simulink model "satsim"  (R2022b)
settings: Solver=VariableStepAuto  StartTime=0.0  StopTime=3600  RelTol=1e-3
InitFcn:
  | run data_initialize.m
StopFcn:
  | figure;
  | subplot(3,1,1);
  | plot(out.t,out.error_anles(:,1));
  | ylabel('yaw(deg)');
  | xlabel('simtime(s)');
  | 
  | subplot(3,1,2);
  | plot(out.t,out.error_anles(:,2));
  | ylabel('pitch(deg)');
  | xlabel('simtime(s)');
  | 
  | subplot(3,1,3);
  | plot(out.t,out.error_anles(:,3));
  | ylabel('roll(deg)');
  | xlabel('simtime(s)');
values from neighbouring files (symbols this model uses):
  Hb0 = IBd*Wb0    [data_initialize.m]
  IBd = [93,-0.07,0;-0.07,80,-0.03;0,-0.03,107]    [data_initialize.m]
  InvIBd = inv(IBd)    [data_initialize.m]
  miu = 398600.44e+9    (= 398600440000000)    [data_initialize.m]    (also in magnetic_Torque.m)
  Qb0 = [1;0;0;0]    [data_initialize.m]
  r0 = 1e+6*[-0.24322284327422;-3.79199144866264;6.32444994784559]    [data_initialize.m]
  T_orbit = 2*pi/Womag    [data_initialize.m]    (also in magnetic_Torque.m)
  v0 = 1e+3*[-1.64209188480826; 6.17220916529869; 3.63756062689151]    [data_initialize.m]
undefined symbols (not defined in the file or in its folder): magnetic_Torque
libraries: sharedutil x4, sharedtransform x2
settings Model: Creator=kuokc  LastModifiedBy=kuokc
settings DebuggingCC: UnderSpecifiedDimensionMsg=warning

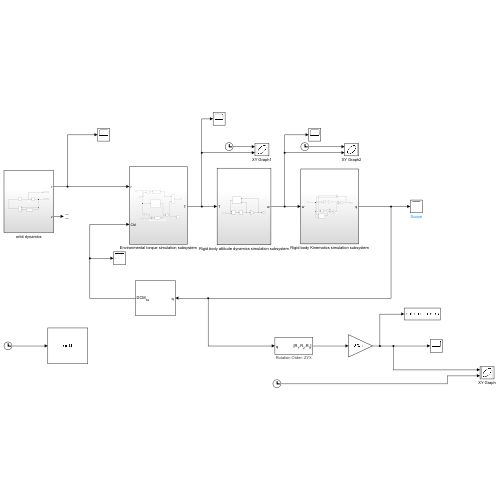
[thumbnail: Simulink's stored preview of the top-level diagram]
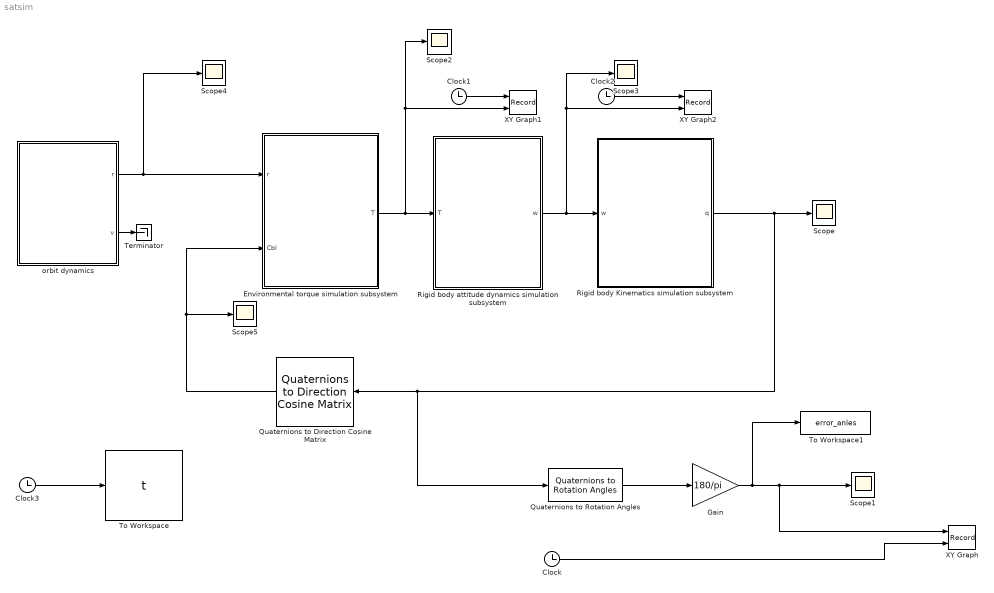
== system satsim ==
  Clock{,1..3} (4 alike) : Clock
  Environmental torque simulation subsystem : Subsystem
  Gain : Gain  Gain=180/pi
  Quaternions to Direction Cosine Matrix : sharedtransform/Quaternions to  Direction Cosine Matrix  aMode=aMode
      settings: LibrarySourceBlock=|
      | aerolibtransform2/Quaternions to
      | Direction Cosine Matrix
  Quaternions to Rotation Angles : sharedtransform/Quaternions to Rotation Angles  rotationOrder=ZYX  aMode=aMode
  Rigid body Kinematics simulation subsystem : Subsystem
  Rigid body attitude dynamics simulation subsystem : Subsystem
  Scope{,1..5} (6 alike) : Scope
  Terminator : Terminator
  To Workspace : ToWorkspace  VariableName=t  SampleTime=-1
  To Workspace1 : ToWorkspace  VariableName=error_anles  SampleTime=-1
  XY Graph : Record  FileSettingsInternal="{\"entries\":[{\"content\":{\"excelSettings\":{\"content\":{},\"type\":\"Streamout.ExcelSettings\"}},\"type\":\"Streamout.FileSettingStorage\",\"uuid\":\"d5935534-3018-4682-9264-9e126ec8adf6\"}],\"packageUris\":[\"http://schema.mathworks.com/mf0/streamout_blocks/R2020a\"],\"version\":\"1.0\"}"  Layout=[1 1]  SignalsInternal="{\"entries\":[{\"content\":{\"signals\":[{\"content\":{\"blockPath\":[\"satsim/XY Graph\"],\"channel\":[],\"dimensions\":[3],\"domain\":\"satsim/XY Graph\",\"hasChildren\":true,\"lineColor\":\"#fe330a\",\"plots\":[],\"port\":1,\"sid\":[\"\"],\"signalID\":166,\"signalName\":\"Gain\"},\"type\":\"RecordBlkView.Signal\",\"uuid\":\"ff8d8c7c-5dc9-4f5c-8804-467ea547fb30\"},{\"content\":{\"blockPath\":[\"satsim/XY Graph\"],\"channel\":[1],\"dimensions\":[3],\"domain\":\"satsim/XY Graph\",\"lineColor\":\"#ff6929\",\"parentID\":166,\"plots\":[1],\"port\":1,\"sid\":[\"\"],\"signalID\":167,\"signalName\":\"Gain\"},\"type\":\"RecordBlkView.Signal\",\"uuid\":\"aac24d3e-19aa-4daa-bfc7-aa7599c39485\"},{\"content\":{\"blockPath\":[\"satsim/XY Graph\"],\"channel\":[],\"dimensions\":[1],\"domain\":\"satsim/XY Graph\",\"lineColor\":\"#139fff\",\"plots\":[1],\"port\":2,\"sid\":[\"\"],\"signalID\":171,\"signalName\":\"Clock\"},\"type\":\"RecordBlkView.Signal\",\"uuid\":\"c5ea15f9-4ec4-4ccd-9c11-f3da415460d7\"},{\"content\":{\"blockPath\":[\"satsim/XY Graph\"],\"channel\":[2],\"dimensions\":[3],\"domain\":\"satsim/XY Graph\",\"lineColor\":\"#7e2f8e\",\"parentID\":166,\"plots\":[1],\"port\":1,\"sid\":[\"\"],\"signalID\":223,\"signalName\":\"Gain\"},\"type\":\"RecordBlkView.Signal\",\"uuid\":\"33786e91-945b-4266-af8d-a53b52915fa5\"},{\"content\":{\"blockPath\":[\"satsim/XY Graph\"],\"channel\":[3],\"dimensions\":[3],\"domain\":\"satsim/XY Graph\",\"lineColor\":\"#77ac30\",\"parentID\":166,\"plots\":[1],\"port\":1,\"sid\":[\"\"],\"signalID\":224,\"signalName\":\"Gain\"},\"type\":\"RecordBlkView.Signal\",\"uuid\":\"7c01fa1b-1002-497a-81b7-3edfb265aba0\"}]},\"type\":\"RecordBlkView.InputSignals\",\"uuid\":\"e2e14102-18f6-4548-bbad-20976a6fad0f\"}],\"packageUris\":[\"http://schema.mathworks.com/mf0/streamout_blocks/R2020a\"],\"version\":\"1.0\"}"  VisualizationBindings="{\"xyplotplugin\":{\"info\":[{\"series\":[{\"bindingParametersList\":[{\"parameter\":\"X-Axis\",\"signalID\":171,\"signalName\":\"Clock\"},{\"parameter\":\"Y-Axis\",\"signalID\":167,\"signalName\":\"Gain(1)\"}],\"seriesID\":65218},{\"bindingParametersList\":[{\"parameter\":\"X-Axis\",\"signalID\":171,\"signalName\":\"Clock\"},{\"parameter\":\"Y-Axis\",\"signalID\":223,\"signalName\":\"Gain(2)\"}],\"seriesID\":37351},{\"bindingParametersList\":[{\"parameter\":\"X-Axis\",\"signalID\":171,\"signalName\":\"Clock\"},{\"parameter\":\"Y-Axis\",\"signalID\":224,\"signalName\":\"Gain(3)\"}],\"seriesID\":18376}],\"subplotID\":1}]}}"  CompatibilityTag=XY
  XY Graph1 : Record  FileSettingsInternal="{\"entries\":[{\"content\":{\"excelSettings\":{\"content\":{},\"type\":\"Streamout.ExcelSettings\"}},\"type\":\"Streamout.FileSettingStorage\",\"uuid\":\"255aa934-7037-4e8a-b86c-47c5749866d0\"}],\"packageUris\":[\"http://schema.mathworks.com/mf0/streamout_blocks/R2020a\"],\"version\":\"1.0\"}"  Layout=[1 1]  SignalsInternal="{\"entries\":[{\"content\":{\"signals\":[{\"content\":{\"blockPath\":[\"satsim/XY Graph1\"],\"channel\":[],\"dimensions\":[1],\"domain\":\"satsim/XY Graph1\",\"lineColor\":\"#139fff\",\"plots\":[1],\"port\":1,\"sid\":[\"\"],\"signalID\":175,\"signalName\":\"Clock1\"},\"type\":\"RecordBlkView.Signal\",\"uuid\":\"f30088d5-5af3-48de-8442-de16e8626a94\"},{\"content\":{\"blockPath\":[\"satsim/XY Graph1\"],\"channel\":[],\"dimensions\":[3],\"domain\":\"satsim/XY Graph1\",\"hasChildren\":true,\"lineColor\":\"#edb120\",\"plots\":[],\"port\":2,\"sid\":[\"\"],\"signalID\":179,\"signalName\":\"Environmental torque simulation subsystem\"},\"type\":\"RecordBlkView.Signal\",\"uuid\":\"edce25b7-b2b4-4c0f-8394-da9e60d165bc\"},{\"content\":{\"blockPath\":[\"satsim/XY Graph1\"],\"channel\":[1],\"dimensions\":[3],\"domain\":\"satsim/XY Graph1\",\"lineColor\":\"#b746ff\",\"parentID\":179,\"plots\":[1],\"port\":2,\"sid\":[\"\"],\"signalID\":180,\"signalName\":\"Environmental torque simulation subsystem\"},\"type\":\"RecordBlkView.Signal\",\"uuid\":\"6268e222-72db-4a7c-9950-fb12145a70e4\"},{\"content\":{\"blockPath\":[\"satsim/XY Graph1\"],\"channel\":[2],\"dimensions\":[3],\"domain\":\"satsim/XY Graph1\",\"lineColor\":\"#4dbeee\",\"parentID\":179,\"plots\":[1],\"port\":2,\"sid\":[\"\"],\"signalID\":225,\"signalName\":\"Environmental torque simulation subsystem\"},\"type\":\"RecordBlkView.Signal\",\"uuid\":\"601717bb-ab46-42cc-a806-3aeeabde5761\"},{\"content\":{\"blockPath\":[\"satsim/XY Graph1\"],\"channel\":[3],\"dimensions\":[3],\"domain\":\"satsim/XY Graph1\",\"lineColor\":\"#a2142f\",\"parentID\":179,\"plots\":[1],\"port\":2,\"sid\":[\"\"],\"signalID\":226,\"signalName\":\"Environmental torque simulation subsystem\"},\"type\":\"RecordBlkView.Signal\",\"uuid\":\"82322a17-9809-4131-ba40-ba05a57ed190\"}]},\"type\":\"RecordBlkView.InputSignals\",\"uuid\":\"6b813904-0c0e-4fcd-a3f5-5389ecdd5549\"}],\"packageUris\":[\"http://schema.mathworks.com/mf0/streamout_blocks/R2020a\"],\"version\":\"1.0\"}"  VisualizationBindings="{\"xyplotplugin\":{\"info\":[{\"series\":[{\"bindingParametersList\":[{\"parameter\":\"X-Axis\",\"signalID\":175,\"signalName\":\"Clock1\"},{\"parameter\":\"Y-Axis\",\"signalID\":225,\"signalName\":\"Environmental torque simulation subsystem(2)\"}],\"seriesID\":232},{\"bindingParametersList\":[{\"parameter\":\"X-Axis\",\"signalID\":175,\"signalName\":\"Clock1\"},{\"parameter\":\"Y-Axis\",\"signalID\":180,\"signalName\":\"Environmental torque simulation subsystem(1)\"}],\"seriesID\":54442},{\"bindingParametersList\":[{\"parameter\":\"X-Axis\",\"signalID\":175,\"signalName\":\"Clock1\"},{\"parameter\":\"Y-Axis\",\"signalID\":226,\"signalName\":\"Environmental torque simulation subsystem(3)\"}],\"seriesID\":10841}],\"subplotID\":1}]}}"  CompatibilityTag=XY
  XY Graph2 : Record  FileSettingsInternal="{\"entries\":[{\"content\":{\"excelSettings\":{\"content\":{},\"type\":\"Streamout.ExcelSettings\"}},\"type\":\"Streamout.FileSettingStorage\",\"uuid\":\"a904b502-5531-4921-b81d-345613b13fcd\"}],\"packageUris\":[\"http://schema.mathworks.com/mf0/streamout_blocks/R2020a\"],\"version\":\"1.0\"}"  Layout=[1 1]  SignalsInternal="{\"entries\":[{\"content\":{\"signals\":[{\"content\":{\"blockPath\":[\"satsim/XY Graph2\"],\"channel\":[],\"dimensions\":[1],\"domain\":\"satsim/XY Graph2\",\"lineColor\":\"#139fff\",\"plots\":[1],\"port\":1,\"sid\":[\"\"],\"signalID\":184,\"signalName\":\"Clock2\"},\"type\":\"RecordBlkView.Signal\",\"uuid\":\"078e9baf-7ef4-4016-bcd0-3751340707a6\"},{\"content\":{\"blockPath\":[\"satsim/XY Graph2\"],\"channel\":[],\"dimensions\":[3],\"domain\":\"satsim/XY Graph2\",\"hasChildren\":true,\"lineColor\":\"#4dbeee\",\"plots\":[],\"port\":2,\"sid\":[\"\"],\"signalID\":188,\"signalName\":\"Rigid body attitude dynamics simulation subsystem\"},\"type\":\"RecordBlkView.Signal\",\"uuid\":\"c9ad4af1-ab2d-4e04-a6fb-069e0a9b0214\"},{\"content\":{\"blockPath\":[\"satsim/XY Graph2\"],\"channel\":[1],\"dimensions\":[3],\"domain\":\"satsim/XY Graph2\",\"lineColor\":\"#b746ff\",\"parentID\":188,\"plots\":[1],\"port\":2,\"sid\":[\"\"],\"signalID\":189,\"signalName\":\"Rigid body attitude dynamics simulation subsystem\"},\"type\":\"RecordBlkView.Signal\",\"uuid\":\"ffc096b0-7673-4870-9807-8de7d9d5d4a3\"},{\"content\":{\"blockPath\":[\"satsim/XY Graph2\"],\"channel\":[2],\"dimensions\":[3],\"domain\":\"satsim/XY Graph2\",\"lineColor\":\"#4dbeee\",\"parentID\":188,\"plots\":[1],\"port\":2,\"sid\":[\"\"],\"signalID\":227,\"signalName\":\"Rigid body attitude dynamics simulation subsystem\"},\"type\":\"RecordBlkView.Signal\",\"uuid\":\"53275a63-6ee4-490c-ab35-1f561b321303\"},{\"content\":{\"blockPath\":[\"satsim/XY Graph2\"],\"channel\":[3],\"dimensions\":[3],\"domain\":\"satsim/XY Graph2\",\"lineColor\":\"#a2142f\",\"parentID\":188,\"plots\":[1],\"port\":2,\"sid\":[\"\"],\"signalID\":228,\"signalName\":\"Rigid body attitude dynamics simulation subsystem\"},\"type\":\"RecordBlkView.Signal\",\"uuid\":\"53a253ef-b50a-41c3-8cb9-5fbddfddb443\"}]},\"type\":\"RecordBlkView.InputSignals\",\"uuid\":\"eac32adb-4985-4d46-95b6-7ca8e99f0a7e\"}],\"packageUris\":[\"http://schema.mathworks.com/mf0/streamout_blocks/R2020a\"],\"version\":\"1.0\"}"  VisualizationBindings="{\"xyplotplugin\":{\"info\":[{\"series\":[{\"bindingParametersList\":[{\"parameter\":\"X-Axis\",\"signalID\":184,\"signalName\":\"Clock2\"},{\"parameter\":\"Y-Axis\",\"signalID\":228,\"signalName\":\"Rigid body attitude dynamics simulation subsystem(3)\"}],\"seriesID\":16914},{\"bindingParametersList\":[{\"parameter\":\"X-Axis\",\"signalID\":184,\"signalName\":\"Clock2\"},{\"parameter\":\"Y-Axis\",\"signalID\":227,\"signalName\":\"Rigid body attitude dynamics simulation subsystem(2)\"}],\"seriesID\":8746},{\"bindingParametersList\":[{\"parameter\":\"X-Axis\",\"signalID\":184,\"signalName\":\"Clock2\"},{\"parameter\":\"Y-Axis\",\"signalID\":189,\"signalName\":\"Rigid body attitude dynamics simulation subsystem(1)\"}],\"seriesID\":5743}],\"subplotID\":1}]}}"  CompatibilityTag=XY
  orbit dynamics : Subsystem
  wires:
  Rigid body attitude dynamics simulation subsystem/1(w) -> XY Graph2/2, Scope3/1, Rigid body Kinematics simulation subsystem/1(w)
  Environmental torque simulation subsystem/1(T) -> XY Graph1/2, Scope2/1, Rigid body attitude dynamics simulation subsystem/1(T)
  orbit dynamics/2(v) -> Terminator/1
  Quaternions to Direction Cosine Matrix/1 -> Scope5/1, Environmental torque simulation subsystem/2(CbI)
  Rigid body Kinematics simulation subsystem/1(q) -> Quaternions to Rotation Angles/1, Quaternions to Direction Cosine Matrix/1, Scope/1
  Quaternions to Rotation Angles/1 -> Gain/1
  Gain/1 -> To Workspace1/1, XY Graph/1, Scope1/1
  Clock/1 -> XY Graph/2
  Clock1/1 -> XY Graph1/1
  Clock2/1 -> XY Graph2/1
  Clock3/1 -> To Workspace/1
  orbit dynamics/1(r) -> Scope4/1, Environmental torque simulation subsystem/1(r)

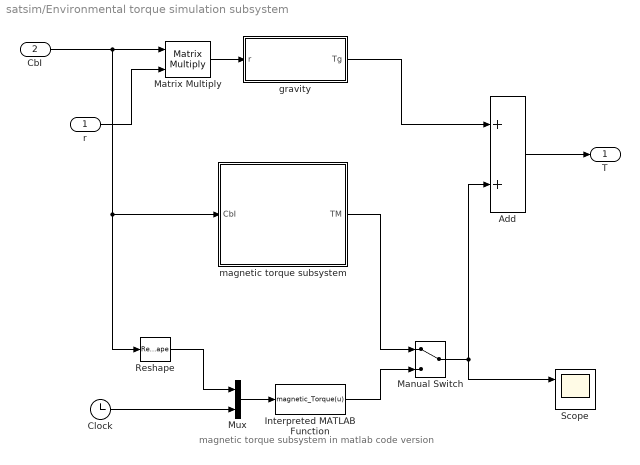
== system satsim/Environmental torque simulation subsystem ==
  note: magnetic torque subsystem in matlab code version
  r : Inport  PortDimensions=3
  CbI : Inport  Port=2
  " gravity" : Subsystem
  Add : Sum
  Clock : Clock
  Interpreted MATLAB Function : MATLABFcn  MATLABFcn=magnetic_Torque(u)  OutputDimensions=3
  Manual Switch : ManualSwitch
  Matrix Multiply : Product  Multiplication=Matrix(*)
  Mux : Mux  Inputs=2
  Reshape : Reshape
  Scope : Scope  NumInputPorts=2
  magnetic torque subsystem : Subsystem
  T : Outport
  wires:
  r/1 -> Matrix Multiply/2
  Matrix Multiply/1 -> " gravity"/1(r)
  " gravity"/1(Tg) -> Add/1
  Add/1 -> T/1
  CbI/1 -> Matrix Multiply/1, magnetic torque subsystem/1(CbI), Reshape/1
  Clock/1 -> Mux/2
  Reshape/1 -> Mux/1
  Mux/1 -> Interpreted MATLAB Function/1
  Interpreted MATLAB Function/1 -> Manual Switch/2
  Manual Switch/1 -> Add/2, Scope/1
  magnetic torque subsystem/1(TM) -> Manual Switch/1

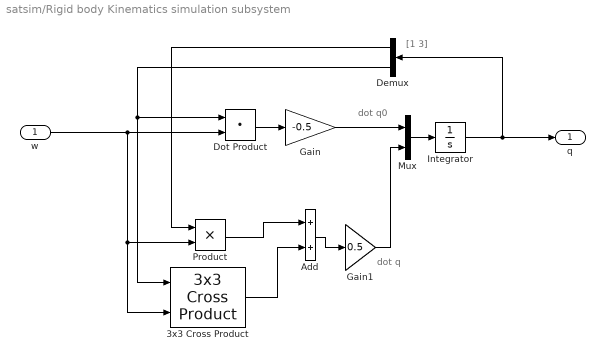
== system satsim/Rigid body Kinematics simulation subsystem ==
  note: [1 3]
  note: dot q
  note: dot q0
  w : Inport  PortDimensions=3
  3x3 Cross Product : sharedutil/3x3 Cross Product  aMode=aMode
      settings: LibrarySourceBlock=aerolibutil/3x3 Cross Product
  Add : Sum
  Demux : Demux  Outputs=2
  Dot Product : DotProduct  OutDataTypeStr=Inherit: Inherit via internal rule
  Gain : Gain  Gain=-0.5
  Gain1 : Gain  Gain=0.5
  Integrator : Integrator  InitialCondition=Qb0
  Mux : Mux  Inputs=2
  Product : Product
  q : Outport
  wires:
  w/1 -> Product/2, 3x3 Cross Product/2, Dot Product/2
  Dot Product/1 -> Gain/1
  Integrator/1 -> Demux/1, q/1
  Mux/1 -> Integrator/1
  Gain/1 -> Mux/1
  Add/1 -> Gain1/1
  Gain1/1 -> Mux/2
  Product/1 -> Add/1
  3x3 Cross Product/1 -> Add/2
  Demux/1 -> Product/1
  Demux/2 -> 3x3 Cross Product/1, Dot Product/1

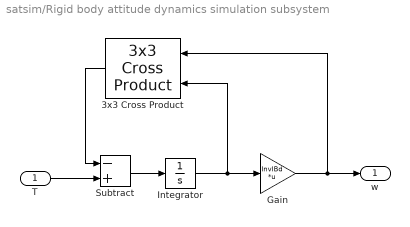
== system satsim/Rigid body attitude dynamics simulation subsystem ==
  T : Inport
  3x3 Cross Product : sharedutil/3x3 Cross Product  aMode=aMode
      settings: LibrarySourceBlock=aerolibutil/3x3 Cross Product
  Gain : Gain  Gain=InvIBd  Multiplication=Matrix(K*u)
  Integrator : Integrator  InitialCondition=Hb0
  Subtract : Sum  Inputs=-+
  w : Outport
  wires:
  T/1 -> Subtract/2
  Subtract/1 -> Integrator/1
  Integrator/1 -> 3x3 Cross Product/2, Gain/1
  3x3 Cross Product/1 -> Subtract/1
  Gain/1 -> 3x3 Cross Product/1, w/1

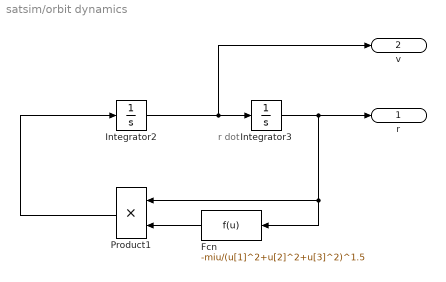
== system satsim/orbit dynamics ==
  note: r dot
  Fcn : Fcn  Expr=-miu/(u[1]^2+u[2]^2+u[3]^2)^1.5
  Integrator2 : Integrator  InitialCondition=v0
  Integrator3 : Integrator  InitialCondition=r0
  Product1 : Product
  r : Outport
  v : Outport  Port=2
  wires:
  Integrator3/1 -> Product1/1, Fcn/1, r/1
  Fcn/1 -> Product1/2
  Product1/1 -> Integrator2/1
  Integrator2/1 -> v/1, Integrator3/1

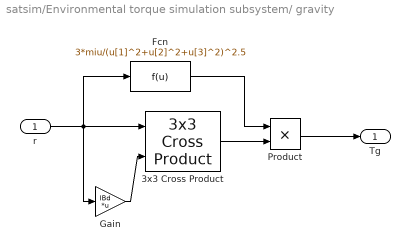
== system satsim/Environmental torque simulation subsystem/ gravity ==
  r : Inport
  3x3 Cross Product : sharedutil/3x3 Cross Product  aMode=aMode
      settings: LibrarySourceBlock=aerolibutil/3x3 Cross Product
  Fcn : Fcn  Expr=3*miu/(u[1]^2+u[2]^2+u[3]^2)^2.5
  Gain : Gain  Gain=IBd  Multiplication=Matrix(K*u)
  Product : Product
  Tg : Outport
  wires:
  r/1 -> Fcn/1, 3x3 Cross Product/1, Gain/1
  Product/1 -> Tg/1
  3x3 Cross Product/1 -> Product/2
  Fcn/1 -> Product/1
  Gain/1 -> 3x3 Cross Product/2

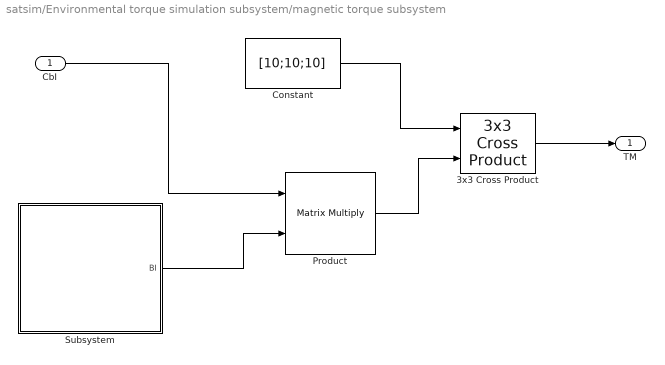
== system satsim/Environmental torque simulation subsystem/magnetic torque subsystem ==
  CbI : Inport
  3x3 Cross Product : sharedutil/3x3 Cross Product  aMode=aMode
      settings: LibrarySourceBlock=aerolibutil/3x3 Cross Product
  Constant : Constant  Value=[10;10;10]
  Product : Product  Multiplication=Matrix(*)
  Subsystem : Subsystem
  TM : Outport
  wires:
  3x3 Cross Product/1 -> TM/1
  Subsystem/1(BI) -> Product/2
  Constant/1 -> 3x3 Cross Product/1
  Product/1 -> 3x3 Cross Product/2
  CbI/1 -> Product/1

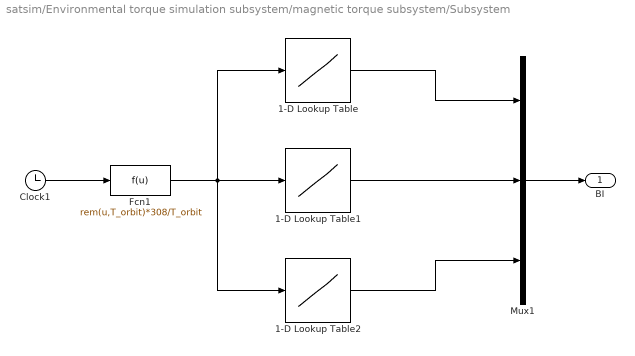
== system satsim/Environmental torque simulation subsystem/magnetic torque subsystem/Subsystem ==
  1-D Lookup Table : Lookup_n-D  NumberOfTableDimensions=1  BreakpointsForDimension1=[1 2 3 4 5 6 7 8 9 10 11 12 13 14 15 16 17 18 19 20 21 22 23 24 25 26 27 28 29 30 31 32 33 34 35 36 37 38 39 40 41 42 43 44 45 46 47 48 49 50 51 52 53 54 55 56 57 58 59 60 61 62 63 64 65 66 67 68 69 70 71 72 73 74 75 76 77 78 79 80 81 82 83 84 85 86 87 88 89 90 91 92 93 94 95 96 97 98 99 100 101 102 103 104 105 106 107 108 109 110 111 112 113 114 115 116 117 118 119 120 121 122 123 124 125 126 127 128 129 130 131 132 133 134 135 136 137 138 139 140 141 142 143 144 145 146 147 148 149 150 151 152 153 154 155 156 157 158 159 160 161 162 163 164 165 166 167 168 169 170 171 172 173 174 175 176 177 178 179 180 181 182 183 184 185 186 187 188 189 190 191 192 193 194 195 196 197 198 199 200 201 202 203 204 205 206 207 208 209 210 211 212 213 214 215 216 217 218 219 220 221 222 223 224 225 226 227 228 229 230 231 232 233 234 235 236 237 238 239 240 241 242 243 244 245 246 247 248 249 250 251 252 253 254 255 256 257 258 259 260 261 262 263 264 265 266 267 268 269 270 271 272 273 274 275 276 277 278 279 280 281 282 283 284 285 286 287 288 289 290 291 292 293 294 295 296 297 298 299 300 301 302 303 304 305 306 307 308]  Table=[-2.55122059735e-05;-2.53831368732e-05;-2.52235856156e-05;-2.50340039571e-05;-2.48149904855e-05;-2.45672896141e-05;-2.42917889233e-05;-2.39895148346e-05;-2.36616266287e-05;-2.33094088488e-05;-2.29342621597e-05;-2.53777161388e-05;-2.51118086265e-05;-2.48212361178e-05;-2.4506733135e-05;-2.41691136071e-05;-2.38092685829e-05;-2.34281630635e-05;-2.30268319106e-05;-2.26063748081e-05;-2.21679502833e-05;-2.17127688231e-05;-2.12420851485e-05;-2.07571897394e-05;-2.02593997327e-05;-1.97500493359e-05;-1.92304799263e-05;-1.87020300159e-05;-1.81660252791e-05;-1.76237688423e-05;-1.70765320346e-05;-1.65255457912e-05;-1.59719928877e-05;-1.54170011619e-05;-1.48616378566e-05;-1.43069051825e-05;-1.37537371709e-05;-1.32029978429e-05;-1.26554806886e-05;-1.21119094065e-05;-1.15729398169e-05;-1.10391628293e-05;-1.05111083076e-05;-9.9892496546e-06;-9.4740089126e-06;-8.9657621649e-06;-8.4648450131e-06;-7.9715579085e-06;-7.4861711209e-06;-7.0089291467e-06;-6.5400543785e-06;-6.0797498887e-06;-5.6282012155e-06;-5.1855770763e-06;-4.7520289788e-06;-4.3276897422e-06;-3.9126709866e-06;-3.5070596917e-06;-3.1109139666e-06;-2.7242582087e-06;-2.3470778625e-06;-1.9793140104e-06;-1.6208580501e-06;-1.2715467158e-06;-9.311577067e-07;-5.994061739e-07;-2.759423012e-07;3.96498102e-08;3.478517774e-07;6.492089552e-07;9.443267491e-07;1.2338651816e-06;1.5185317245e-06;1.7990724643e-06;2.0762617185e-06;2.3508902742e-06;2.6237524583e-06;2.8956322887e-06;3.1672889751e-06;3.439442053e-06;3.712756446e-06;3.9878277898e-06;4.2651684793e-06;4.5451951611e-06;4.8282186893e-06;5.1144374378e-06;5.4039337333e-06;5.6966715987e-06;5.9924941754e-06;6.2911218023e-06;6.5921534619e-06;6.895072788e-06;7.199257676e-06;7.5039922277e-06;7.8084805091e-06;8.1118620334e-06;8.4132288451e-06;8.7116439108e-06;9.0061604131e-06;9.2958414958e-06;9.5797799999e-06;9.857117732e-06;1.01270638228e-05;1.03889117529e-05;1.06420546553e-05;1.08859985423e-05;1.11203731537e-05;1.13449401783e-05;1.15595986644e-05;1.17643875001e-05;1.19594849177e-05;1.21452050435e-05;1.23219915885e-05;1.24904088417e-05;1.26511301904e-05;1.28049244517e-05;1.29526403445e-05;1.30951894767e-05;1.32335282498e-05;1.33686391035e-05;1.3501511532e-05;1.36331233009e-05;1.37644222797e-05;1.38963092803e-05;1.40296222578e-05;1.41651221878e-05;1.43034808824e-05;1.44452709521e-05;1.45909580612e-05;1.47408955592e-05;1.48953215088e-05;1.50543580702e-05;1.52180131402e-05;1.53861840909e-05;1.55586634062e-05;1.57351459714e-05;1.59152377411e-05;1.60984654855e-05;1.62842873042e-05;1.64721035914e-05;1.6661268144e-05;1.6851099117e-05;1.70408895585e-05;1.7229917283e-05;1.74174538811e-05;1.76027727076e-05;1.77851557294e-05;1.79638991672e-05;1.81383179065e-05;1.83077487023e-05;1.84715522384e-05;1.86291141439e-05;1.87798450982e-05;1.8923180179e-05;1.90585776294e-05;1.91855172246e-05;1.9303498425e-05;1.94120384921e-05;1.95106707367e-05;1.95989430434e-05;1.96764167947e-05;1.97426662892e-05;1.97972787144e-05;1.98398547032e-05;1.987000947e-05;1.98873744888e-05;1.98915996478e-05;1.98823557895e-05;1.98593375226e-05;1.98222661818e-05;1.97708927966e-05;1.97050009356e-05;1.96244092915e-05;1.95289738866e-05;1.94185897961e-05;1.92931923062e-05;1.9152757454e-05;1.8997301922e-05;1.88268822956e-05;1.86415937194e-05;1.84415680214e-05;1.82269714009e-05;1.79980018006e-05;1.77548861022e-05;1.74978772986e-05;1.72272518013e-05;1.69433070433e-05;1.66463595264e-05;1.633674345e-05;1.60148100341e-05;1.56809276211e-05;1.53354826087e-05;1.49788812273e-05;1.46115521343e-05;1.4233949759e-05;1.38465582863e-05;1.34498961328e-05;1.30445207308e-05;1.26310334053e-05;1.22100841079e-05;1.17823757529e-05;1.13486678951e-05;1.09097794898e-05;1.04665904877e-05;1.00200420368e-05;9.5711350951e-06;9.1209272945e-06;8.6705279423e-06;8.2210910989e-06;7.7738067254e-06;7.3298899548e-06;6.8905685985e-06;6.4570690618e-06;6.0306008938e-06;5.6123402526e-06;5.2034126074e-06;4.8048750396e-06;4.4176985294e-06;4.0427506318e-06;3.6807789539e-06;3.332395837e-06;2.9980646316e-06;2.6780879248e-06;2.3725980409e-06 ...(+1522 chars)]  InterpMethod=Linear Lagrange  InternalRulePriority=Speed  RndMeth=Simplest
  1-D Lookup Table1 : Lookup_n-D  NumberOfTableDimensions=1  BreakpointsForDimension1=[1 2 3 4 5 6 7 8 9 10 11 12 13 14 15 16 17 18 19 20 21 22 23 24 25 26 27 28 29 30 31 32 33 34 35 36 37 38 39 40 41 42 43 44 45 46 47 48 49 50 51 52 53 54 55 56 57 58 59 60 61 62 63 64 65 66 67 68 69 70 71 72 73 74 75 76 77 78 79 80 81 82 83 84 85 86 87 88 89 90 91 92 93 94 95 96 97 98 99 100 101 102 103 104 105 106 107 108 109 110 111 112 113 114 115 116 117 118 119 120 121 122 123 124 125 126 127 128 129 130 131 132 133 134 135 136 137 138 139 140 141 142 143 144 145 146 147 148 149 150 151 152 153 154 155 156 157 158 159 160 161 162 163 164 165 166 167 168 169 170 171 172 173 174 175 176 177 178 179 180 181 182 183 184 185 186 187 188 189 190 191 192 193 194 195 196 197 198 199 200 201 202 203 204 205 206 207 208 209 210 211 212 213 214 215 216 217 218 219 220 221 222 223 224 225 226 227 228 229 230 231 232 233 234 235 236 237 238 239 240 241 242 243 244 245 246 247 248 249 250 251 252 253 254 255 256 257 258 259 260 261 262 263 264 265 266 267 268 269 270 271 272 273 274 275 276 277 278 279 280 281 282 283 284 285 286 287 288 289 290 291 292 293 294 295 296 297 298 299 300 301 302 303 304 305 306 307 308]  Table=[5.3943408503e-06;5.451945977e-06;5.5099840032e-06;5.5686785233e-06;5.6282573934e-06;5.6889497235e-06;5.7509828588e-06;5.8145793907e-06;5.8799542372e-06;5.94731183e-06;6.0168434444e-06;4.7087073539e-06;4.7375390485e-06;4.7708591853e-06;4.8088064599e-06;4.8514966586e-06;4.8990214362e-06;4.9514473778e-06;5.0088153506e-06;5.0711401447e-06;5.1384103978e-06;5.2105887907e-06;5.2876124951e-06;5.3693938514e-06;5.4558212485e-06;5.5467601785e-06;5.6420544324e-06;5.7415274061e-06;5.8449834862e-06;5.9522094832e-06;6.0629760863e-06;6.1770393143e-06;6.2941419425e-06;6.4140148876e-06;6.5363785406e-06;6.6609440389e-06;6.7874144761e-06;6.9154860506e-06;7.0448491591e-06;7.1751894438e-06;7.3061888062e-06;7.4375263993e-06;7.5688796147e-06;7.6999250787e-06;7.8303396713e-06;7.9598015803e-06;8.0879914017e-06;8.2145932914e-06;8.3392961734e-06;8.4617950021e-06;8.5817920749e-06;8.6989983852e-06;8.8131350026e-06;8.9239344627e-06;9.0311421467e-06;9.1345176268e-06;9.2338359525e-06;9.3288888511e-06;9.419485817e-06;9.5054550626e-06;9.5866443079e-06;9.6629213878e-06;9.734174658e-06;9.8003131876e-06;9.8612667281e-06;9.9169854571e-06;9.9674394974e-06;1.00126182194e-05;1.00525293401e-05;1.00871978374e-05;1.01166646999e-05;1.01409855412e-05;1.01602291052e-05;1.01744756932e-05;1.01838155438e-05;1.01883471949e-05;1.01881758554e-05;1.01834118183e-05;1.01741689501e-05;1.01605633118e-05;1.01427120155e-05;1.01207324874e-05;1.00947423786e-05;1.00648603053e-05;1.00312071818e-05;9.9939070975e-06;9.9530862011e-06;9.9088692678e-06;9.8613762245e-06;9.8107215627e-06;9.7570167285e-06;9.7003730361e-06;9.6409033075e-06;9.5787223099e-06;9.5139467591e-06;9.446695351e-06;9.3770888947e-06;9.3052504682e-06;9.231305516e-06;9.1553818467e-06;9.0776095136e-06;8.9981205846e-06;8.9170488093e-06;8.8345292003e-06;8.7506975478e-06;8.6656898872e-06;8.579641942e-06;8.4926885672e-06;8.4049632128e-06;8.3165974329e-06;8.2277204577e-06;8.1384588481e-06;8.0489362448e-06;7.959273222e-06;7.8695872515e-06;7.7799927742e-06;7.6906013771e-06;7.601522061e-06;7.5128615872e-06;7.4247248807e-06;7.3372154673e-06;7.2504359192e-06;7.1644882791e-06;7.0794744365e-06;6.9954964252e-06;6.9126566177e-06;6.8310577904e-06;6.7508030411e-06;6.6719955419e-06;6.5947381187e-06;6.5191326531e-06;6.4452793097e-06;6.3732755997e-06;6.3032152958e-06;6.2351872235e-06;6.1692739572e-06;6.1055504556e-06;6.0440826767e-06;5.9849262129e-06;5.9281249907e-06;5.8737100809e-06;5.8216986606e-06;5.7720931695e-06;5.7248806981e-06;5.6800326375e-06;5.6375046193e-06;5.5972367606e-06;5.5591542262e-06;5.5231681068e-06;5.489176605e-06;5.4570665126e-06;5.4267149498e-06;5.3979913337e-06;5.3707595304e-06;5.344880143e-06;5.3202128808e-06;5.2966189492e-06;5.2739634018e-06;5.2521173932e-06;5.2309602719e-06;5.2103814582e-06;5.1902820553e-06;5.1705761482e-06;5.1511917544e-06;5.1320713964e-06;5.1131722811e-06;5.0944660755e-06;5.0759382847e-06;5.0575872465e-06;5.0394227671e-06;5.0214644348e-06;5.003739656e-06;4.986281466e-06;4.9691261747e-06;4.9523109111e-06;4.9358711344e-06;4.9198381802e-06;4.9042369106e-06;4.8890835334e-06;4.8743836521e-06;4.860130602e-06;4.8463041197e-06;4.8328693849e-06;4.8197764647e-06;4.806960176e-06;4.794340375e-06;4.7818226683e-06;4.7692995309e-06;4.7566518035e-06;4.7437505335e-06;4.7304591157e-06;4.7166356775e-06;4.7021356526e-06;4.686814478e-06;4.6705303493e-06;4.6531469674e-06;4.63453621e-06;4.6145806653e-06;4.5931759682e-06;4.5702328856e-06;4.5456791045e-06;4.5194606848e-06;4.4915431466e-06;4.4619121735e-06;4.4305739199e-06;4.397554925e-06;4.3629016395e-06;4.3266795869e-06;4.2889721838e-06;4.2498792552e-06;4.2095152853e-06;4.1680074485e-06;4.1254934727e-06;4.0821193841e-06;4.0380371891e-06;3.993402544e-06;3.9483724649e-06;3.9031031248e-06;3.8577477823e-06;3.8124548809e-06;3.7673663524e-06;3.7226161512e-06;3.6783290388e-06;3.6346196337e-06;3.5915917292e-06;3.5493378784e-06;3.5079392358e-06;3.4674656332e-06;3.4279758596e-06;3.3895181e-06;3.3521304707e-06;3.3158415803e-06;3.2806710468e-06;3.2466299676e-06;3.2137215296e-06 ...(+1235 chars)]  InterpMethod=Linear Lagrange  InternalRulePriority=Speed  RndMeth=Simplest
  1-D Lookup Table2 : Lookup_n-D  NumberOfTableDimensions=1  BreakpointsForDimension1=[1 2 3 4 5 6 7 8 9 10 11 12 13 14 15 16 17 18 19 20 21 22 23 24 25 26 27 28 29 30 31 32 33 34 35 36 37 38 39 40 41 42 43 44 45 46 47 48 49 50 51 52 53 54 55 56 57 58 59 60 61 62 63 64 65 66 67 68 69 70 71 72 73 74 75 76 77 78 79 80 81 82 83 84 85 86 87 88 89 90 91 92 93 94 95 96 97 98 99 100 101 102 103 104 105 106 107 108 109 110 111 112 113 114 115 116 117 118 119 120 121 122 123 124 125 126 127 128 129 130 131 132 133 134 135 136 137 138 139 140 141 142 143 144 145 146 147 148 149 150 151 152 153 154 155 156 157 158 159 160 161 162 163 164 165 166 167 168 169 170 171 172 173 174 175 176 177 178 179 180 181 182 183 184 185 186 187 188 189 190 191 192 193 194 195 196 197 198 199 200 201 202 203 204 205 206 207 208 209 210 211 212 213 214 215 216 217 218 219 220 221 222 223 224 225 226 227 228 229 230 231 232 233 234 235 236 237 238 239 240 241 242 243 244 245 246 247 248 249 250 251 252 253 254 255 256 257 258 259 260 261 262 263 264 265 266 267 268 269 270 271 272 273 274 275 276 277 278 279 280 281 282 283 284 285 286 287 288 289 290 291 292 293 294 295 296 297 298 299 300 301 302 303 304 305 306 307 308]  Table=[-4.961439257e-07;-1.7357945627e-06;-2.9641301952e-06;-4.1787546858e-06;-5.3773102582e-06;-6.5574946903e-06;-7.7170784681e-06;-8.8539216579e-06;-9.9659902549e-06;-1.10513717659e-05;-1.21082897926e-05;-1.07596031871e-05;-1.19663117919e-05;-1.31540841681e-05;-1.43212395271e-05;-1.54661580047e-05;-1.65872892927e-05;-1.76831612531e-05;-1.87523883599e-05;-1.9793679804e-05;-2.08058470856e-05;-2.17878109213e-05;-2.27386072909e-05;-2.36573924672e-05;-2.4543446881e-05;-2.53961777023e-05;-2.62151200432e-05;-2.69999367213e-05;-2.77504165572e-05;-2.84664712199e-05;-2.91481306702e-05;-2.9795537292e-05;-3.04089388397e-05;-3.09886803604e-05;-3.15351952826e-05;-3.20489958841e-05;-3.25306633719e-05;-3.29808378148e-05;-3.34002081747e-05;-3.3789502674e-05;-3.41494797257e-05;-3.44809196325e-05;-3.47846172293e-05;-3.50613756146e-05;-3.53120010732e-05;-3.5537299251e-05;-3.57380725984e-05;-3.59151190492e-05;-3.60692318605e-05;-3.62012004921e-05;-3.63118123662e-05;-3.64018553145e-05;-3.64721204888e-05;-3.6523405496e-05;-3.65565175014e-05;-3.65722760444e-05;-3.65715153167e-05;-3.65550856665e-05;-3.65238541185e-05;-3.64787037311e-05;-3.64205316514e-05;-3.63502457737e-05;-3.62687599591e-05;-3.61769878252e-05;-3.60758351712e-05;-3.59661911555e-05;-3.58489184001e-05;-3.57248422365e-05;-3.55947393605e-05;-3.54593261896e-05;-3.53192472517e-05;-3.51750639473e-05;-3.50272440387e-05;-3.48761522148e-05;-3.47220420694e-05;-3.45650498037e-05;-3.44051899343e-05;-3.42423532401e-05;-3.40763071332e-05;-3.39066985782e-05;-3.37330596218e-05;-3.35548155254e-05;-3.33712954267e-05;-3.31817453818e-05;-3.2985343579e-05;-3.27812174457e-05;-3.2568462316e-05;-3.23461612772e-05;-3.21134057694e-05;-3.18693164854e-05;-3.16130640971e-05;-3.13438893281e-05;-3.10611218966e-05;-3.07641978724e-05;-3.04526750188e-05;-3.01262457343e-05;-2.97847472587e-05;-2.94281688698e-05;-2.90566558662e-05;-2.86705102053e-05;-2.82701877458e-05;-2.78562921223e-05;-2.74295653638e-05;-2.69908754425e-05;-2.65412010168e-05;-2.60816136974e-05;-2.56132582285e-05;-2.51373310223e-05;-2.46550575288e-05;-2.41676689455e-05;-2.3676378791e-05;-2.31823598623e-05;-2.26867220887e-05;-2.2190491769e-05;-2.16945926394e-05;-2.11998291766e-05;-2.07068724787e-05;-2.02162490038e-05;-1.97283323719e-05;-1.92433383615e-05;-1.87613231513e-05;-1.82821847803e-05;-1.78056677228e-05;-1.73313703996e-05;-1.68587553841e-05;-1.63871619986e-05;-1.59158209498e-05;-1.54438706114e-05;-1.4970374534e-05;-1.44943397477e-05;-1.40147354172e-05;-1.35305114203e-05;-1.30406164366e-05;-1.25440151684e-05;-1.20397043513e-05;-1.15267272633e-05;-1.10041864944e-05;-1.04712547979e-05;-9.9271839069e-06;-9.3713112624e-06;-8.8030646592e-06;-8.2219648772e-06;-7.6276264162e-06;-7.0197565007e-06;-6.3981525622e-06;-5.7626984337e-06;-5.1133595172e-06;-4.4501771918e-06;-3.7732627377e-06;-3.0827910362e-06;-2.378994299e-06;-1.6621560457e-06;-9.326055259e-07;-1.907127403e-07;5.631158218e-07;1.3284406569e-06;2.1047918994e-06;2.891671166e-06;3.6885526385e-06;4.4948834719e-06;5.3100836404e-06;6.1335453563e-06;6.9646322169e-06;7.8026782354e-06;8.6469869184e-06;9.4968305421e-06;1.03514497645e-05;1.12100536923e-05;1.20718204943e-05;1.29358986213e-05;1.38014086643e-05;1.46674458453e-05;1.55330831024e-05;1.63973747028e-05;1.72593602838e-05;1.81180692049e-05;1.89725250707e-05;1.98217502781e-05;2.06647704333e-05;2.15006184922e-05;2.23283384835e-05;2.31469886973e-05;2.39556442413e-05;2.47533989007e-05;2.55393662693e-05;2.63126801566e-05;2.70724943159e-05;2.78179815729e-05;2.8548332473e-05;2.9262753597e-05;2.9960465722e-05;3.06407020238e-05;3.13027065341e-05;3.19457330653e-05;3.25690448158e-05;3.31719148536e-05;3.37536276528e-05;3.43134818275e-05;3.48507941692e-05;3.53649050469e-05;3.58551851792e-05;3.63210437348e-05;3.67619376591e-05;3.71773820727e-05;3.75669615308e-05;3.79303418856e-05;3.82672824514e-05;3.85776481335e-05;3.8861421161e-05;3.91187120439e-05;3.93497693738e-05;3.9554988093e-05;3.97349158791e-05;3.9890257321e-05;4.00218756065e-05;4.01307914933e-05 ...(+1641 chars)]  InterpMethod=Linear Lagrange  InternalRulePriority=Speed  RndMeth=Simplest
  Clock1 : Clock
  Fcn1 : Fcn  Expr=rem(u,T_orbit)*308/T_orbit
  Mux1 : Mux  Inputs=3
  BI : Outport
  wires:
  1-D Lookup Table/1 -> Mux1/1
  1-D Lookup Table2/1 -> Mux1/3
  Clock1/1 -> Fcn1/1
  Fcn1/1 -> 1-D Lookup Table2/1, 1-D Lookup Table/1, 1-D Lookup Table1/1
  Mux1/1 -> BI/1
  1-D Lookup Table1/1 -> Mux1/2
